simulink model "Model_aircraft_simple"  (R2024b)
settings: Solver=ode45  StartTime=0.0  StopTime=T_fin  RelTol=1e-10  EnableMultiTasking=on
values from neighbouring files (symbols this model uses):
  Euler_0 = [0; 0; 0]    [Main_simple.m]    (also in Script_trim_AI.m = x_trim(7:9))
  g = 9.81    [Main_simple.m]
  pqr_0 = [0; 0; 0]    [Main_simple.m]
  Ref_altitude = 0    [Main_simple.m]
  rho_0 = 1.293    [Main_simple.m]
  Tot_mom_inertia = diag([0.0494,0.0583,0.1012])    [Main_simple.m]
  Total_mass = 0.573    [Main_simple.m]
  u_0 = [0; 0; 0; 0]    [Main_simple.m]    (also in Script_trim_AI.m = u_0+u_trim)
  uvw_0 = [12.37 ;0; 0]    [Main_simple.m]    (also in Script_trim_AI.m = x_trim(4:6))
libraries: Library_simple_model x7
settings Model: Creator=Drago  LastModifiedBy=gregor
settings SolverCC: AlgebraicLoopSolver=TrustRegion
settings DataIOCC: LimitDataPoints=on  SaveFormat=Array
settings OptimizationCC: LifeSpan=inf
settings DebuggingCC: UnconnectedInputMsg=warning  UnconnectedOutputMsg=warning  UnconnectedLineMsg=warning  InitInArrayFormatMsg=none  SFUnexpectedBacktrackingDiag=warning  SFNoUnconditionalDefaultTransitionDiag=warning  SFExecutionAtInitializationDiag=none  ArithmeticOperatorsInVariantConditions=warning
settings HardwareCC: ProdBitPerPointer=32  ProdBitPerSizeT=32  ProdBitPerPtrDiffT=32  ProdLargestAtomicFloat=None  ProdIntDivRoundTo=Undefined  ProdEndianess=Unspecified  ProdWordSize=32  ProdHWDeviceType=32-bit Generic
settings ModelReferenceCC: EnableRefExpFcnMdlSchedulingChecks=on  PropagateSignalLabelsOutOfModel=off
settings SFSimCC: SimUseLocalCustomCode=off  CustomCodeUndefinedFunction=UseInterfaceOnly
settings RTWCC: RTWUseLocalCustomCode=off  GPUComputeCapability=3.5  DLArmComputeVersion=19.05
settings CodeAppCC: StateflowObjectComments=on
settings GRTTargetCC: TargetLangStandard=C89/C90 (ANSI)
settings ConfigComp: CovMetricSettings=dw  CovSaveCumulativeToWorkspaceVar=on  CovSaveSingleToWorkspaceVar=on  CovExternalEMLEnable=off  CovSFcnEnable=off

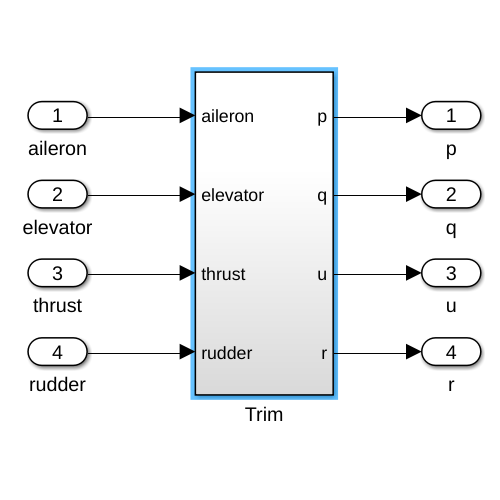
[thumbnail: Simulink's stored preview of the top-level diagram]
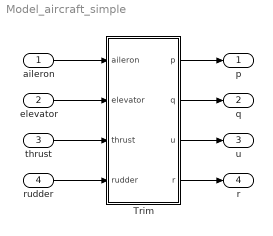
== system Model_aircraft_simple ==
  aileron : Inport
  elevator : Inport  Port=2
  thrust : Inport  Port=3
  rudder : Inport  Port=4
  Trim : Subsystem
  p : Outport
  q : Outport  Port=2
  u : Outport  Port=3
  r : Outport  Port=4
  wires:
  aileron/1 -> Trim/1(aileron)
  elevator/1 -> Trim/2(elevator)
  thrust/1 -> Trim/3(thrust)
  rudder/1 -> Trim/4(rudder)
  Trim/1(p) -> p/1
  Trim/2(q) -> q/1
  Trim/3(u) -> u/1
  Trim/4(r) -> r/1

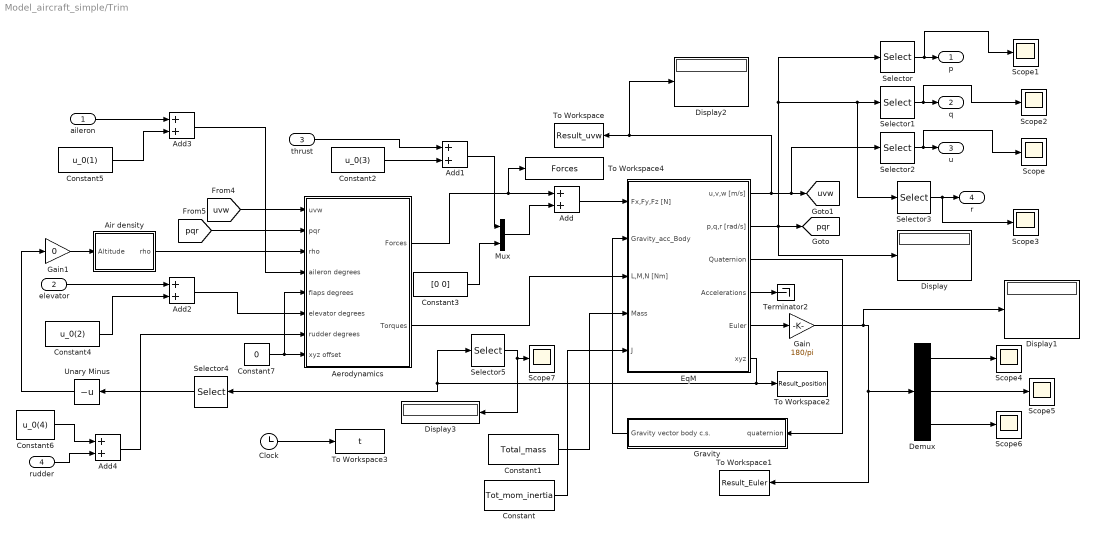
== system Model_aircraft_simple/Trim ==
  aileron : Inport
  elevator : Inport  Port=2
  thrust : Inport  Port=3
  rudder : Inport  Port=4
  Add{,1..4} (5 alike) : Sum
  "Aerodynamics " : Subsystem
  Air density : Subsystem
  Clock : Clock
  Constant : Constant  Value=Tot_mom_inertia
  Constant1 : Constant  Value=Total_mass
  Constant2 : Constant  Value=u_0(3)
  Constant3 : Constant  Value=[0 0]
  Constant4 : Constant  Value=u_0(2)
  Constant5 : Constant  Value=u_0(1)
  Constant6 : Constant  Value=u_0(4)
  Constant7 : Constant  Value=0
  Demux : Demux  Outputs=3
  Display{,1..3} (4 alike) : Display
  EqM : Subsystem
  Gain : Gain  Gain=180/pi
  Gain1 : Gain  Gain=0
  Gravity : Subsystem
  Mux : Mux  Inputs=2
  Scope{,1..7} (8 alike) : Scope
  Selector : Selector  InputPortWidth=3  IndexOptions=Index vector (dialog)  Indices=1  OutputSizes=1
  Selector1 : Selector  InputPortWidth=3  IndexOptions=Index vector (dialog)  Indices=2  OutputSizes=1
  Selector2 : Selector  InputPortWidth=3  IndexOptions=Index vector (dialog)  Indices=1  OutputSizes=1
  Selector3 : Selector  InputPortWidth=3  IndexOptions=Index vector (dialog)  Indices=3  OutputSizes=1
  Selector4 : Selector  InputPortWidth=3  IndexOptions=Index vector (dialog)  Indices=3  OutputSizes=1
  Selector5 : Selector  InputPortWidth=3  IndexOptions=Index vector (dialog)  Indices=3  OutputSizes=1
  Terminator2 : Terminator
  To Workspace : ToWorkspace  VariableName=Result_uvw  SampleTime=0.2
  To Workspace1 : ToWorkspace  VariableName=Result_Euler  SampleTime=0.2
  To Workspace2 : ToWorkspace  VariableName=Result_position  SampleTime=0.2
  To Workspace3 : ToWorkspace  VariableName=t  SampleTime=0.2
  To Workspace4 : ToWorkspace  VariableName=Forces  SampleTime=0.2
  Unary Minus : UnaryMinus
  p : Outport
  q : Outport  Port=2
  u : Outport  Port=3
  r : Outport  Port=4
  tag scope: pqr=global, uvw=global
  wires:
  Add1/1 -> Mux/1
  Gain/1 -> Display1/1, Demux/1, To Workspace1/1
  EqM/4(Accelerations) -> Terminator2/1
  Air density/1(rho) -> "Aerodynamics "/3(rho)
  EqM/2(p,q,r [rad/s]) -> Display/1, Selector3/1, Selector1/1, Selector/1, [pqr]
  Gravity/1(Gravity vector body c.s.) -> EqM/2(Gravity_acc_Body)
  EqM/3(Quaternion) -> Gravity/1(quaternion)
  [uvw] -> "Aerodynamics "/1(uvw)
  Add/1 -> EqM/1(Fx,Fy,Fz [N])
  "Aerodynamics "/2(Torques) -> EqM/3(L,M,N [Nm])
  "Aerodynamics "/1(Forces) -> To Workspace4/1, Add/1
  Constant1/1 -> EqM/4(Mass)
  EqM/1(u,v,w [m/s]) -> Display2/1, To Workspace/1, Selector2/1, [uvw]
  Constant/1 -> EqM/5(J)
  [pqr] -> "Aerodynamics "/2(pqr)
  EqM/5(Euler) -> Gain/1
  Constant3/1 -> Mux/2
  rudder/1 -> Add4/2
  Selector4/1 -> Unary Minus/1
  Mux/1 -> Add/2
  Add3/1 -> "Aerodynamics "/4(aileron degrees)
  Constant2/1 -> Add1/2
  aileron/1 -> Add3/1
  elevator/1 -> Add2/1
  Constant4/1 -> Add2/2
  Constant5/1 -> Add3/2
  Add4/1 -> "Aerodynamics "/7(rudder degrees)
  thrust/1 -> Add1/1
  Add2/1 -> "Aerodynamics "/6(elevator degrees)
  EqM/6(xyz) -> Selector4/1, Selector5/1, To Workspace2/1
  Constant6/1 -> Add4/1
  Clock/1 -> To Workspace3/1
  Constant7/1 -> "Aerodynamics "/5(flaps degrees), "Aerodynamics "/8(xyz offset)
  Selector/1 -> Scope1/1, p/1
  Selector1/1 -> Scope2/1, q/1
  Selector2/1 -> Scope/1, u/1
  Selector3/1 -> Scope3/1, r/1
  Unary Minus/1 -> Gain1/1
  Demux/1 -> Scope4/1
  Demux/2 -> Scope5/1
  Demux/3 -> Scope6/1
  Selector5/1 -> Display3/1, Scope7/1
  Gain1/1 -> Air density/1(Altitude)

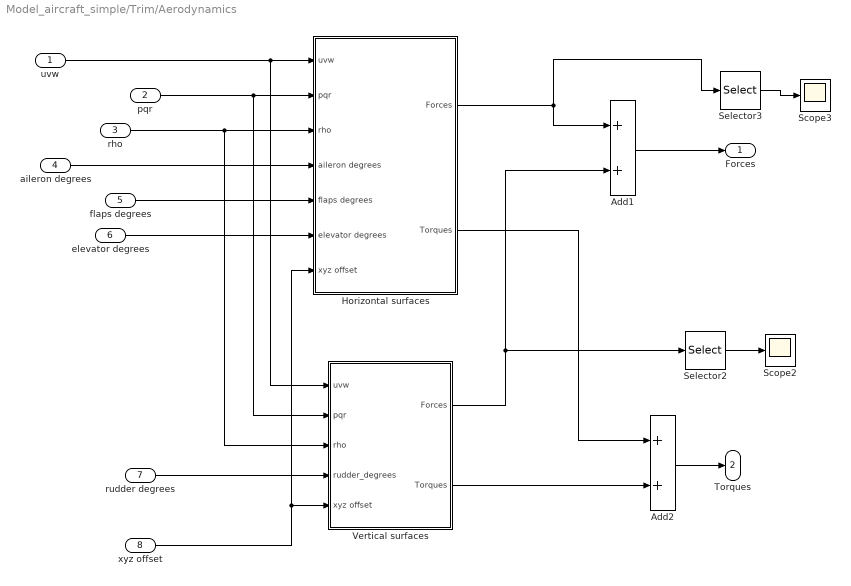
== system Model_aircraft_simple/Trim/Aerodynamics  ==
  uvw : Inport
  pqr : Inport  Port=2
  rho : Inport  Port=3
  aileron degrees : Inport  Port=4
  flaps degrees : Inport  Port=5
  elevator degrees : Inport  Port=6
  rudder degrees : Inport  Port=7
  xyz offset : Inport  Port=8
  Add1 : Sum
  Add2 : Sum
  Horizontal surfaces : Subsystem
  Scope2 : Scope
  Scope3 : Scope
  Selector2 : Selector  InputPortWidth=3  IndexOptions=Index vector (dialog)  Indices=[1 ]  OutputSizes=1
  Selector3 : Selector  InputPortWidth=3  IndexOptions=Index vector (dialog)  Indices=[1 ]  OutputSizes=1
  Vertical surfaces : Subsystem
  Forces : Outport
  Torques : Outport  Port=2
  wires:
  elevator degrees/1 -> Horizontal surfaces/6(elevator degrees)
  aileron degrees/1 -> Horizontal surfaces/4(aileron degrees)
  xyz offset/1 -> Horizontal surfaces/7(xyz offset), Vertical surfaces/5(xyz offset)
  rho/1 -> Vertical surfaces/3(rho), Horizontal surfaces/3(rho)
  pqr/1 -> Vertical surfaces/2(pqr), Horizontal surfaces/2(pqr)
  flaps degrees/1 -> Horizontal surfaces/5(flaps degrees)
  uvw/1 -> Vertical surfaces/1(uvw), Horizontal surfaces/1(uvw)
  Add2/1 -> Torques/1
  Horizontal surfaces/1(Forces) -> Selector3/1, Add1/1
  Add1/1 -> Forces/1
  Vertical surfaces/1(Forces) -> Selector2/1, Add1/2
  Horizontal surfaces/2(Torques) -> Add2/1
  rudder degrees/1 -> Vertical surfaces/4(rudder_degrees)
  Vertical surfaces/2(Torques) -> Add2/2
  Selector2/1 -> Scope2/1
  Selector3/1 -> Scope3/1

== system Model_aircraft_simple/Trim/Air density ==
  Altitude : Inport
  Gain : Gain  Gain=rho_0
  exp(-h/8000) : Fcn  Expr=exp(-u(1)/8000)
  rho : Outport
  wires:
  Gain/1 -> rho/1
  Altitude/1 -> exp(-h/8000)/1
  exp(-h/8000)/1 -> Gain/1

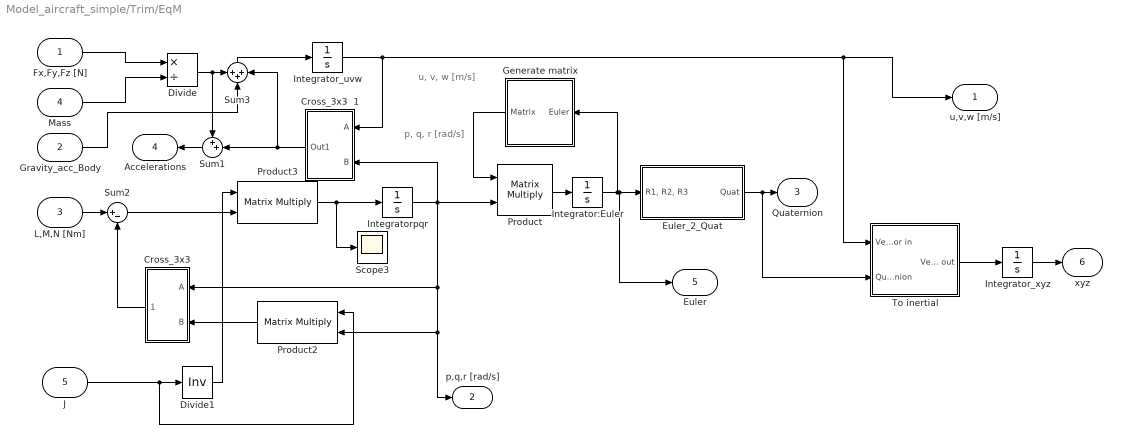
== system Model_aircraft_simple/Trim/EqM ==
  note: u, v, w [m/s]
  note: p, q, r [rad/s]
  Fx,Fy,Fz [N] : Inport
  Gravity_acc_Body : Inport  Port=2
  L,M,N [Nm] : Inport  Port=3
  Mass : Inport  Port=4
  J : Inport  Port=5
  Cross_3x3 : Subsystem
  Cross_3x3  1 : Subsystem
  Divide : Product  Inputs=*/
  Divide1 : Product  Inputs=/  Multiplication=Matrix(*)
  Euler_2_Quat : Subsystem
  Generate matrix : Subsystem
  Integrator:Euler : Integrator  InitialCondition=Euler_0  ZeroCross=off
  Integrator_uvw : Integrator  InitialCondition=uvw_0  ZeroCross=off
  Integrator_xyz : Integrator  InitialCondition=[0 0 -Ref_altitude]  ZeroCross=off
  Integratorpqr : Integrator  InitialCondition=pqr_0  ZeroCross=off
  Product : Product  Multiplication=Matrix(*)
  Product2 : Product  Multiplication=Matrix(*)
  Product3 : Product  Multiplication=Matrix(*)
  Scope3 : Scope
  Sum1 : Sum  Inputs=++|
  Sum2 : Sum  Inputs=|+-
  Sum3 : Sum  Inputs=+++
  To inertial : Subsystem
  u,v,w [m/s] : Outport
  p,q,r [rad/s] : Outport  Port=2
  Quaternion : Outport  Port=3
  Accelerations : Outport  Port=4
  Euler : Outport  Port=5
  xyz : Outport  Port=6
  wires:
  L,M,N [Nm]/1 -> Sum2/1
  Fx,Fy,Fz [N]/1 -> Divide/1
  Euler_2_Quat/1(Quat) -> To inertial/2(Quaternion), Quaternion/1
  Product2/1 -> Cross_3x3/2(B)
  Product3/1 -> Scope3/1, Integratorpqr/1
  Sum2/1 -> Product3/2
  Sum3/1 -> Integrator_uvw/1
  Integrator_uvw/1 -> Cross_3x3  1/1(A), To inertial/1(Vector in), u,v,w [m/s]/1
  Integratorpqr/1 -> Product/2, Cross_3x3  1/2(B), Product2/2, p,q,r [rad/s]/1, Cross_3x3/1(A)
  Cross_3x3/1(Out1) -> Sum2/2
  Cross_3x3  1/1(Out1) -> Sum3/3, Sum1/2
  Gravity_acc_Body/1 -> Sum3/2
  Divide/1 -> Sum1/1, Sum3/1
  Sum1/1 -> Accelerations/1
  Mass/1 -> Divide/2
  J/1 -> Product2/1, Divide1/1
  Divide1/1 -> Product3/1
  To inertial/1(Vector out) -> Integrator_xyz/1
  Integrator_xyz/1 -> xyz/1
  Product/1 -> Integrator:Euler/1
  Generate matrix/1(Matrix) -> Product/1
  Integrator:Euler/1 -> Generate matrix/1("Euler "), Euler_2_Quat/1("R1, R2, R3"), Euler/1

== system Model_aircraft_simple/Trim/Gravity ==
  quaternion : Inport
  Gravitational force : Constant  Value=[0 0 g]
  Inertial_2_body1 : Subsystem
  Gravity vector body c.s. : Outport
  wires:
  Gravitational force/1 -> Inertial_2_body1/1(Vector in)
  quaternion/1 -> Inertial_2_body1/2(Quaternion)
  Inertial_2_body1/1(Vector out) -> Gravity vector body c.s./1

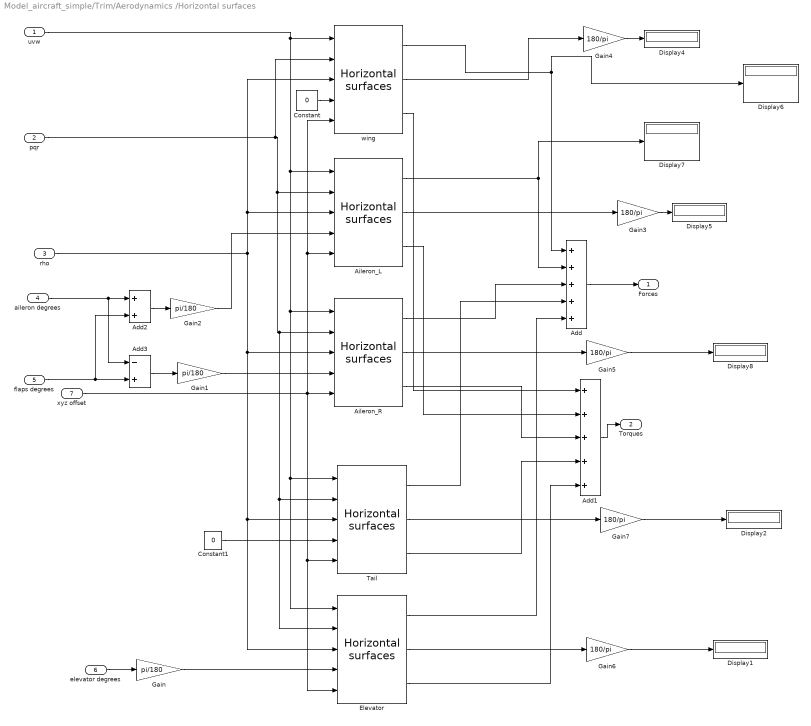
== system Model_aircraft_simple/Trim/Aerodynamics /Horizontal surfaces ==
  uvw : Inport
  pqr : Inport  Port=2
  rho : Inport  Port=3
  aileron degrees : Inport  Port=4
  flaps degrees : Inport  Port=5
  elevator degrees : Inport  Port=6
  xyz offset : Inport  Port=7
  Add : Sum  Inputs=+++++
  Add1 : Sum  Inputs=+++++
  Add2 : Sum
  Add3 : Sum  Inputs=-+
  Aileron_L : Library_simple_model/Horizontal surfaces  xyz_Aero=xyz_aileron_L  S_Wing=S__aileron_L  Alpha_0=Alpha_0_aileron_L  Alpha_param_Vector=Alpha_param_vector_aileron_L  CL_param_Vector=CL_param_vector_aileron_L  CD_param_Vector=CD_param_vector_aileron_L
  Aileron_R : Library_simple_model/Horizontal surfaces  xyz_Aero=xyz_aileron_R  S_Wing=S__aileron_R  Alpha_0=Alpha_0_aileron_R  Alpha_param_Vector=Alpha_param_vector_aileron_R  CL_param_Vector=CL_param_vector_aileron_R  CD_param_Vector=CD_param_vector_aileron_R
  Constant : Constant  Value=0
  Constant1 : Constant  Value=0
  Display{1..2,4..8} (7 alike) : Display
  Elevator : Library_simple_model/Horizontal surfaces  xyz_Aero=xyz_elevator  S_Wing=S_elevator  Alpha_0=Alpha_0_elevator  Alpha_param_Vector=Alpha_param_vector_elevator  CL_param_Vector=CL_param_vector_elevator  CD_param_Vector=CD_param_vector_elevator
  Gain : Gain  Gain=pi/180
  Gain1 : Gain  Gain=pi/180
  Gain2 : Gain  Gain=pi/180
  Gain{3..7} (5 alike) : Gain  Gain=180/pi
  Tail : Library_simple_model/Horizontal surfaces  xyz_Aero=xyz_horiz_stabilizer  S_Wing=S_horiz_stabilizer  Alpha_0=Alpha_0_horiz_stabilizer  Alpha_param_Vector=Alpha_param_vector_horiz_stabilizer  CL_param_Vector=CL_param_vector_horiz_stabilizer  CD_param_Vector=CD_param_vector_horiz_stabilizer
  wing : Library_simple_model/Horizontal surfaces  xyz_Aero=xyz_wing  S_Wing=S_wing  Alpha_0=Alpha_0_wing  Alpha_param_Vector=Alpha_param_vector_wing  CL_param_Vector=CL_param_vector_wing  CD_param_Vector=CD_param_vector_wing
  Forces : Outport
  Torques : Outport  Port=2
  wires:
  Add1/1 -> Torques/1
  Aileron_R/3 -> Add1/3
  wing/3 -> Add1/1
  pqr/1 -> wing/2, Elevator/2, Tail/2, Aileron_R/2, Aileron_L/2
  aileron degrees/1 -> Add3/1, Add2/1
  elevator degrees/1 -> Gain/1
  Aileron_L/1 -> Display7/1, Add/2
  wing/1 -> Display6/1, Add/1
  Aileron_R/1 -> Add/3
  rho/1 -> Elevator/3, Tail/3, Aileron_R/3, Aileron_L/3, wing/3
  uvw/1 -> wing/1, Elevator/1, Tail/1, Aileron_R/1, Aileron_L/1
  Gain1/1 -> Aileron_R/4
  Add3/1 -> Gain1/1
  Gain2/1 -> Aileron_L/4
  flaps degrees/1 -> Add2/2, Add3/2
  Add2/1 -> Gain2/1
  Add/1 -> Forces/1
  Aileron_L/3 -> Add1/2
  xyz offset/1 -> Elevator/5, Tail/5, Aileron_R/5, Aileron_L/5, wing/5
  wing/2 -> Gain4/1
  Aileron_L/2 -> Gain3/1
  Gain3/1 -> Display5/1
  Gain4/1 -> Display4/1
  Aileron_R/2 -> Gain5/1
  Gain5/1 -> Display8/1
  Constant/1 -> wing/4
  Tail/3 -> Add1/4
  Tail/1 -> Add/4
  Gain/1 -> Elevator/4
  Constant1/1 -> Tail/4
  Elevator/3 -> Add1/5
  Elevator/1 -> Add/5
  Gain6/1 -> Display1/1
  Elevator/2 -> Gain6/1
  Gain7/1 -> Display2/1
  Tail/2 -> Gain7/1

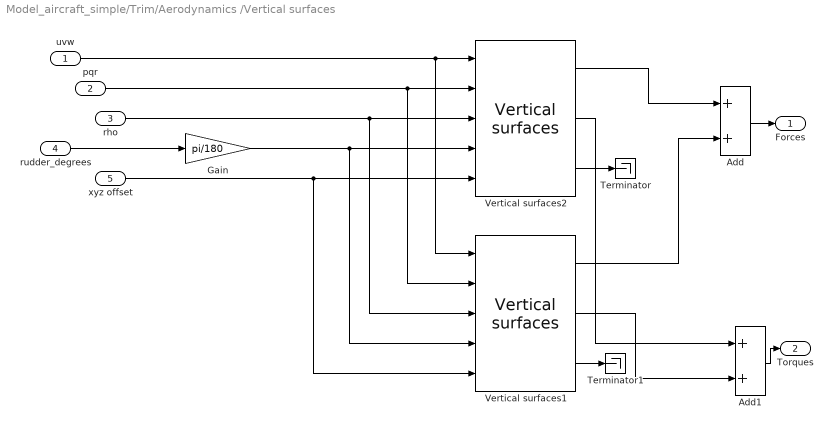
== system Model_aircraft_simple/Trim/Aerodynamics /Vertical surfaces ==
  uvw : Inport
  pqr : Inport  Port=2
  rho : Inport  Port=3
  rudder_degrees : Inport  Port=4
  xyz offset : Inport  Port=5
  Add : Sum
  Add1 : Sum
  Gain : Gain  Gain=pi/180
  Terminator : Terminator
  Terminator1 : Terminator
  Vertical surfaces1 : Library_simple_model/Vertical surfaces  xyzbody_Vert_stab=xyz_rudder  S_Body_Vert_stab=S_rudder  beta_param_Vert_stab_param=Beta_param_vector_rudder  CY_Vert_stab_param=CY_param_vector_rudder  CD_Vert_stab_param=CD_param_vector_rudder
  Vertical surfaces2 : Library_simple_model/Vertical surfaces  xyzbody_Vert_stab=xyz_vert_stabilizer  S_Body_Vert_stab=S_vert_stabilizer  beta_param_Vert_stab_param=Beta_param_vector_vert_stabilizer  CY_Vert_stab_param=CY_param_vector_vert_stabilizer  CD_Vert_stab_param=CD_param_vector_vert_stabilizer
  Forces : Outport
  Torques : Outport  Port=2
  wires:
  pqr/1 -> Vertical surfaces1/2, Vertical surfaces2/2
  rho/1 -> Vertical surfaces1/3, Vertical surfaces2/3
  Vertical surfaces2/3 -> Terminator/1
  xyz offset/1 -> Vertical surfaces1/5, Vertical surfaces2/5
  rudder_degrees/1 -> Gain/1
  uvw/1 -> Vertical surfaces1/1, Vertical surfaces2/1
  Vertical surfaces1/3 -> Terminator1/1
  Add1/1 -> Torques/1
  Vertical surfaces2/1 -> Add/1
  Vertical surfaces1/1 -> Add/2
  Vertical surfaces2/2 -> Add1/1
  Vertical surfaces1/2 -> Add1/2
  Add/1 -> Forces/1
  Gain/1 -> Vertical surfaces1/4, Vertical surfaces2/4

== system Model_aircraft_simple/Trim/EqM/Cross_3x3 ==
  A : Inport
  B : Inport  Port=2
  Subsystem : Subsystem
  Subsystem1 : Subsystem
  Sum2 : Sum  Inputs=+|-  InputSameDT=on  SaturateOnIntegerOverflow=on  OutDataTypeStr=Inherit: Same as first input
  Out1 : Outport
  wires:
  B/1 -> Subsystem/2(B1), Subsystem1/2(B1)
  Subsystem1/1(Out2) -> Sum2/2
  Subsystem/1(Out2) -> Sum2/1
  Sum2/1 -> Out1/1
  A/1 -> Subsystem1/1(A1), Subsystem/1(A1)

== system Model_aircraft_simple/Trim/EqM/Cross_3x3  1 ==
  A : Inport
  B : Inport  Port=2
  Subsystem : Subsystem
  Subsystem1 : Subsystem
  Sum2 : Sum  Inputs=+|-  InputSameDT=on  SaturateOnIntegerOverflow=on  OutDataTypeStr=Inherit: Same as first input
  Out1 : Outport
  wires:
  B/1 -> Subsystem/2(B1), Subsystem1/2(B1)
  Subsystem1/1(Out2) -> Sum2/2
  Subsystem/1(Out2) -> Sum2/1
  Sum2/1 -> Out1/1
  A/1 -> Subsystem1/1(A1), Subsystem/1(A1)

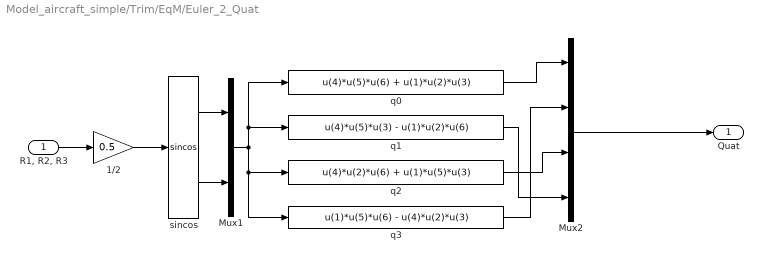
== system Model_aircraft_simple/Trim/EqM/Euler_2_Quat ==
  "R1, R2, R3" : Inport
  1/2 : Gain  Gain=0.5  SaturateOnIntegerOverflow=on  OutDataTypeStr=Inherit: Same as input  ParamDataTypeStr=Inherit: Same as input
  Mux1 : Mux  Inputs=2
  Mux2 : Mux
  q0 : Fcn  Expr=u(4)*u(5)*u(6) + u(1)*u(2)*u(3)
  q1 : Fcn  Expr=u(4)*u(5)*u(3) - u(1)*u(2)*u(6)
  q2 : Fcn  Expr=u(4)*u(2)*u(6) + u(1)*u(5)*u(3)
  q3 : Fcn  Expr=u(1)*u(5)*u(6) - u(4)*u(2)*u(3)
  sincos : Trigonometry  Operator=sincos
  Quat : Outport  InitialOutput=0
  wires:
  q1/1 -> Mux2/4
  sincos/2 -> Mux1/2
  q2/1 -> Mux2/3
  sincos/1 -> Mux1/1
  q0/1 -> Mux2/1
  Mux1/1 -> q0/1, q1/1, q2/1, q3/1
  1/2/1 -> sincos/1
  Mux2/1 -> Quat/1
  q3/1 -> Mux2/2
  "R1, R2, R3"/1 -> 1/2/1

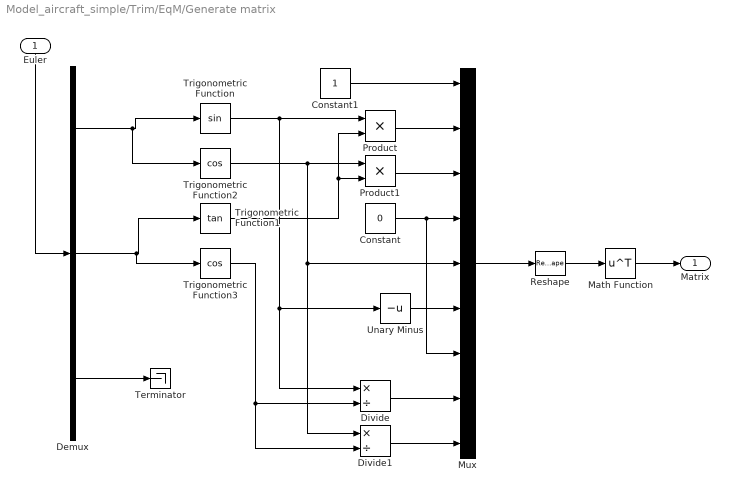
== system Model_aircraft_simple/Trim/EqM/Generate matrix ==
  "Euler " : Inport
  Constant : Constant  Value=0
  Constant1 : Constant
  Demux : Demux  Outputs=3
  Divide : Product  Inputs=*/
  Divide1 : Product  Inputs=*/
  Math Function : Math  Operator=transpose  SignedPower=on
  Mux : Mux  Inputs=9
  Product : Product
  Product1 : Product
  Reshape : Reshape  OutputDimensionality=Customize  OutputDimensions=[3,3]
  Terminator : Terminator
  Trigonometric Function : Trigonometry
  Trigonometric Function1 : Trigonometry  Operator=tan
  Trigonometric Function2 : Trigonometry  Operator=cos
  Trigonometric Function3 : Trigonometry  Operator=cos
  Unary Minus : UnaryMinus
  Matrix : Outport
  wires:
  Demux/1 -> Trigonometric Function2/1, Trigonometric Function/1
  Demux/3 -> Terminator/1
  "Euler "/1 -> Demux/1
  Demux/2 -> Trigonometric Function3/1, Trigonometric Function1/1
  Mux/1 -> Reshape/1
  Product/1 -> Mux/2
  Trigonometric Function/1 -> Divide/1, Unary Minus/1, Product/1
  Trigonometric Function1/1 -> Product1/2, Product/2
  Product1/1 -> Mux/3
  Trigonometric Function2/1 -> Divide1/1, Mux/5, Product1/1
  Unary Minus/1 -> Mux/6
  Constant/1 -> Mux/7, Mux/4
  Divide/1 -> Mux/8
  Divide1/1 -> Mux/9
  Trigonometric Function3/1 -> Divide/2, Divide1/2
  Reshape/1 -> Math Function/1
  Constant1/1 -> Mux/1
  Math Function/1 -> Matrix/1

== system Model_aircraft_simple/Trim/EqM/To inertial ==
  note: To inertial
  Vector in : Inport
  Quaternion : Inport  Port=2
  Conjugate quaternion : Subsystem
  Product of quaternions1 : Subsystem
  Product of quaternions2 : Subsystem
  Quaternion _2_vector : Subsystem
  Vector_2_ quaternion : Subsystem
  Vector out : Outport
  wires:
  Product of quaternions2/1(Out1) -> Product of quaternions1/1(In1)
  Vector_2_ quaternion/1(Out1) -> Product of quaternions2/2(In2)
  Conjugate quaternion/1(Out1) -> Product of quaternions1/2(In2)
  Product of quaternions1/1(Out1) -> Quaternion _2_vector/1(In1)
  Vector in/1 -> Vector_2_ quaternion/1(In1)
  Quaternion/1 -> Conjugate quaternion/1(In1), Product of quaternions2/1(In1)
  Quaternion _2_vector/1(Out1) -> Vector out/1

== system Model_aircraft_simple/Trim/Gravity/Inertial_2_body1 ==
  Vector in : Inport
  Quaternion : Inport  Port=2
  Conjugate quaternion : Subsystem
  Product of quaternions1 : Subsystem
  Product of quaternions2 : Subsystem
  Quaternion _2_vector : Subsystem
  Vector_2_ quaternion : Subsystem
  Vector out : Outport
  wires:
  Product of quaternions2/1(Out1) -> Product of quaternions1/1(In1)
  Vector_2_ quaternion/1(Out1) -> Product of quaternions2/2(In2)
  Product of quaternions1/1(Out1) -> Quaternion _2_vector/1(In1)
  Vector in/1 -> Vector_2_ quaternion/1(In1)
  Quaternion/1 -> Conjugate quaternion/1(In1), Product of quaternions1/2(In2)
  Quaternion _2_vector/1(Out1) -> Vector out/1
  Conjugate quaternion/1(Out1) -> Product of quaternions2/1(In1)

== system Model_aircraft_simple/Trim/EqM/Cross_3x3/Subsystem ==
  A1 : Inport
  B1 : Inport  Port=2
  Demux : Demux  Outputs=3
  Demux1 : Demux  Outputs=3
  Mux : Mux  Inputs=3
  i x j : Product  InputSameDT=on  SaturateOnIntegerOverflow=on  OutDataTypeStr=Inherit: Same as first input
  j x k : Product  InputSameDT=on  SaturateOnIntegerOverflow=on  OutDataTypeStr=Inherit: Same as first input
  k x i : Product  InputSameDT=on  SaturateOnIntegerOverflow=on  OutDataTypeStr=Inherit: Same as first input
  Out2 : Outport
  wires:
  k x i/1 -> Mux/2
  Demux1/2 -> i x j/2
  Demux1/3 -> j x k/2
  Demux1/1 -> k x i/2
  Demux/3 -> k x i/1
  Mux/1 -> Out2/1
  Demux/2 -> j x k/1
  j x k/1 -> Mux/1
  i x j/1 -> Mux/3
  B1/1 -> Demux1/1
  Demux/1 -> i x j/1
  A1/1 -> Demux/1

== system Model_aircraft_simple/Trim/EqM/Cross_3x3/Subsystem1 ==
  A1 : Inport
  B1 : Inport  Port=2
  Demux : Demux  Outputs=3
  Demux1 : Demux  Outputs=3
  Mux : Mux  Inputs=3
  i x k : Product  InputSameDT=on  SaturateOnIntegerOverflow=on  OutDataTypeStr=Inherit: Same as first input
  j x i : Product  InputSameDT=on  SaturateOnIntegerOverflow=on  OutDataTypeStr=Inherit: Same as first input
  k x j : Product  InputSameDT=on  SaturateOnIntegerOverflow=on  OutDataTypeStr=Inherit: Same as first input
  Out2 : Outport
  wires:
  j x i/1 -> Mux/3
  i x k/1 -> Mux/2
  k x j/1 -> Mux/1
  Mux/1 -> Out2/1
  Demux1/1 -> j x i/2
  Demux/2 -> j x i/1
  Demux1/3 -> i x k/2
  Demux/1 -> i x k/1
  Demux/3 -> k x j/1
  Demux1/2 -> k x j/2
  B1/1 -> Demux1/1
  A1/1 -> Demux/1

== system Model_aircraft_simple/Trim/EqM/Cross_3x3  1/Subsystem ==
  A1 : Inport
  B1 : Inport  Port=2
  Demux : Demux  Outputs=3
  Demux1 : Demux  Outputs=3
  Mux : Mux  Inputs=3
  i x j : Product  InputSameDT=on  SaturateOnIntegerOverflow=on  OutDataTypeStr=Inherit: Same as first input
  j x k : Product  InputSameDT=on  SaturateOnIntegerOverflow=on  OutDataTypeStr=Inherit: Same as first input
  k x i : Product  InputSameDT=on  SaturateOnIntegerOverflow=on  OutDataTypeStr=Inherit: Same as first input
  Out2 : Outport
  wires:
  k x i/1 -> Mux/2
  Demux1/2 -> i x j/2
  Demux1/3 -> j x k/2
  Demux1/1 -> k x i/2
  Demux/3 -> k x i/1
  Mux/1 -> Out2/1
  Demux/2 -> j x k/1
  j x k/1 -> Mux/1
  i x j/1 -> Mux/3
  B1/1 -> Demux1/1
  Demux/1 -> i x j/1
  A1/1 -> Demux/1

== system Model_aircraft_simple/Trim/EqM/Cross_3x3  1/Subsystem1 ==
  A1 : Inport
  B1 : Inport  Port=2
  Demux : Demux  Outputs=3
  Demux1 : Demux  Outputs=3
  Mux : Mux  Inputs=3
  i x k : Product  InputSameDT=on  SaturateOnIntegerOverflow=on  OutDataTypeStr=Inherit: Same as first input
  j x i : Product  InputSameDT=on  SaturateOnIntegerOverflow=on  OutDataTypeStr=Inherit: Same as first input
  k x j : Product  InputSameDT=on  SaturateOnIntegerOverflow=on  OutDataTypeStr=Inherit: Same as first input
  Out2 : Outport
  wires:
  j x i/1 -> Mux/3
  i x k/1 -> Mux/2
  k x j/1 -> Mux/1
  Mux/1 -> Out2/1
  Demux1/1 -> j x i/2
  Demux/2 -> j x i/1
  Demux1/3 -> i x k/2
  Demux/1 -> i x k/1
  Demux/3 -> k x j/1
  Demux1/2 -> k x j/2
  B1/1 -> Demux1/1
  A1/1 -> Demux/1

== system Model_aircraft_simple/Trim/EqM/To inertial/Conjugate quaternion ==
  In1 : Inport
  Demux1 : Demux
  Mux1 : Mux
  Unary Minus1 : UnaryMinus
  Unary Minus2 : UnaryMinus
  Unary Minus3 : UnaryMinus
  Out1 : Outport
  wires:
  Demux1/1 -> Mux1/1
  Unary Minus1/1 -> Mux1/2
  Unary Minus2/1 -> Mux1/3
  Unary Minus3/1 -> Mux1/4
  Demux1/2 -> Unary Minus1/1
  Demux1/3 -> Unary Minus2/1
  Demux1/4 -> Unary Minus3/1
  In1/1 -> Demux1/1
  Mux1/1 -> Out1/1

== system Model_aircraft_simple/Trim/EqM/To inertial/Product of quaternions1 ==
  In1 : Inport
  In2 : Inport  Port=2
  Mux : Mux
  q0 : Subsystem
  q1 : Subsystem
  q2 : Subsystem
  q3 : Subsystem
  Out1 : Outport
  wires:
  q0/1(q0) -> Mux/1
  q1/1(q1) -> Mux/2
  q2/1(q2) -> Mux/3
  q3/1(q3) -> Mux/4
  In1/1 -> q3/1(q), q2/1(q), q1/1(q), q0/1(q)
  In2/1 -> q1/2(r), q2/2(r), q3/2(r), q0/2(r)
  Mux/1 -> Out1/1

== system Model_aircraft_simple/Trim/EqM/To inertial/Product of quaternions2 ==
  In1 : Inport
  In2 : Inport  Port=2
  Mux : Mux
  q0 : Subsystem
  q1 : Subsystem
  q2 : Subsystem
  q3 : Subsystem
  Out1 : Outport
  wires:
  q0/1(q0) -> Mux/1
  q1/1(q1) -> Mux/2
  q2/1(q2) -> Mux/3
  q3/1(q3) -> Mux/4
  In1/1 -> q3/1(q), q2/1(q), q1/1(q), q0/1(q)
  In2/1 -> q1/2(r), q2/2(r), q3/2(r), q0/2(r)
  Mux/1 -> Out1/1

== system Model_aircraft_simple/Trim/EqM/To inertial/Quaternion _2_vector ==
  In1 : Inport
  Demux1 : Demux
  Mux1 : Mux  Inputs=3
  Terminator2 : Terminator
  Out1 : Outport
  wires:
  Demux1/2 -> Mux1/1
  Demux1/3 -> Mux1/2
  Demux1/4 -> Mux1/3
  Demux1/1 -> Terminator2/1
  In1/1 -> Demux1/1
  Mux1/1 -> Out1/1

== system Model_aircraft_simple/Trim/EqM/To inertial/Vector_2_ quaternion ==
  note: Vector_2_quaternion
  In1 : Inport
  Constant2 : Constant  Value=0
  Mux : Mux  Inputs=2
  Out1 : Outport
  wires:
  Constant2/1 -> Mux/1
  In1/1 -> Mux/2
  Mux/1 -> Out1/1

== system Model_aircraft_simple/Trim/Gravity/Inertial_2_body1/Conjugate quaternion ==
  In1 : Inport
  Demux1 : Demux
  Mux1 : Mux
  Unary Minus1 : UnaryMinus
  Unary Minus2 : UnaryMinus
  Unary Minus3 : UnaryMinus
  Out1 : Outport
  wires:
  Demux1/1 -> Mux1/1
  Unary Minus1/1 -> Mux1/2
  Unary Minus2/1 -> Mux1/3
  Unary Minus3/1 -> Mux1/4
  Demux1/2 -> Unary Minus1/1
  Demux1/3 -> Unary Minus2/1
  Demux1/4 -> Unary Minus3/1
  In1/1 -> Demux1/1
  Mux1/1 -> Out1/1

== system Model_aircraft_simple/Trim/Gravity/Inertial_2_body1/Product of quaternions1 ==
  In1 : Inport
  In2 : Inport  Port=2
  Mux : Mux
  q0 : Subsystem
  q1 : Subsystem
  q2 : Subsystem
  q3 : Subsystem
  Out1 : Outport
  wires:
  Mux/1 -> Out1/1
  In2/1 -> q0/2(r), q3/2(r), q2/2(r), q1/2(r)
  In1/1 -> q0/1(q), q1/1(q), q2/1(q), q3/1(q)
  q3/1(q3) -> Mux/4
  q2/1(q2) -> Mux/3
  q1/1(q1) -> Mux/2
  q0/1(q0) -> Mux/1

== system Model_aircraft_simple/Trim/Gravity/Inertial_2_body1/Product of quaternions2 ==
  In1 : Inport
  In2 : Inport  Port=2
  Mux : Mux
  q0 : Subsystem
  q1 : Subsystem
  q2 : Subsystem
  q3 : Subsystem
  Out1 : Outport
  wires:
  q0/1(q0) -> Mux/1
  q1/1(q1) -> Mux/2
  q2/1(q2) -> Mux/3
  q3/1(q3) -> Mux/4
  In1/1 -> q3/1(q), q2/1(q), q1/1(q), q0/1(q)
  In2/1 -> q1/2(r), q2/2(r), q3/2(r), q0/2(r)
  Mux/1 -> Out1/1

== system Model_aircraft_simple/Trim/Gravity/Inertial_2_body1/Quaternion _2_vector ==
  In1 : Inport
  Demux1 : Demux
  Mux1 : Mux  Inputs=3
  Terminator2 : Terminator
  Out1 : Outport
  wires:
  Demux1/2 -> Mux1/1
  Demux1/3 -> Mux1/2
  Demux1/4 -> Mux1/3
  Demux1/1 -> Terminator2/1
  In1/1 -> Demux1/1
  Mux1/1 -> Out1/1

== system Model_aircraft_simple/Trim/Gravity/Inertial_2_body1/Vector_2_ quaternion ==
  In1 : Inport
  Constant2 : Constant  Value=0
  Mux : Mux  Inputs=2
  Out1 : Outport
  wires:
  Constant2/1 -> Mux/1
  In1/1 -> Mux/2
  Mux/1 -> Out1/1

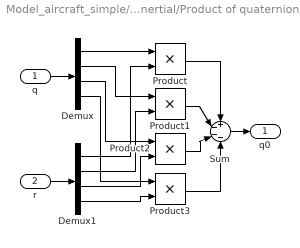
== system Model_aircraft_simple/Trim/EqM/To inertial/Product of quaternions1/q0 ==
  q : Inport
  r : Inport  Port=2
  Demux : Demux
  Demux1 : Demux
  Product{,1..3} (4 alike) : Product  RndMeth=Zero
  Sum : Sum  Inputs=+---
  q0 : Outport
  wires:
  q/1 -> Demux/1
  r/1 -> Demux1/1
  Demux/1 -> Product/1
  Demux1/1 -> Product/2
  Demux/2 -> Product1/1
  Demux1/2 -> Product1/2
  Demux/3 -> Product2/1
  Demux1/3 -> Product2/2
  Demux1/4 -> Product3/2
  Demux/4 -> Product3/1
  Product/1 -> Sum/1
  Product1/1 -> Sum/2
  Product3/1 -> Sum/4
  Sum/1 -> q0/1
  Product2/1 -> Sum/3

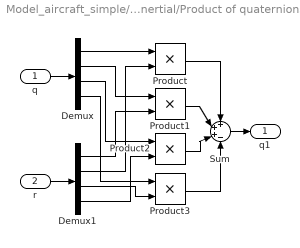
== system Model_aircraft_simple/Trim/EqM/To inertial/Product of quaternions1/q1 ==
  q : Inport
  r : Inport  Port=2
  Demux : Demux
  Demux1 : Demux
  Product{,1..3} (4 alike) : Product  RndMeth=Zero
  Sum : Sum  Inputs=+++-
  q1 : Outport
  wires:
  Product2/1 -> Sum/3
  Sum/1 -> q1/1
  Product3/1 -> Sum/4
  Product1/1 -> Sum/2
  Product/1 -> Sum/1
  Demux/4 -> Product3/1
  Demux/3 -> Product2/1
  Demux/2 -> Product1/1
  Demux/1 -> Product/1
  r/1 -> Demux1/1
  q/1 -> Demux/1
  Demux1/2 -> Product/2
  Demux1/1 -> Product1/2
  Demux1/4 -> Product2/2
  Demux1/3 -> Product3/2

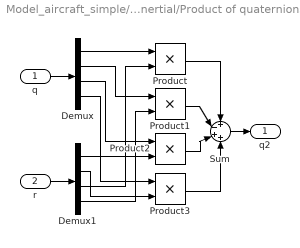
== system Model_aircraft_simple/Trim/EqM/To inertial/Product of quaternions1/q2 ==
  q : Inport
  r : Inport  Port=2
  Demux : Demux
  Demux1 : Demux
  Product{,1..3} (4 alike) : Product  RndMeth=Zero
  Sum : Sum  Inputs=+-++
  q2 : Outport
  wires:
  q/1 -> Demux/1
  r/1 -> Demux1/1
  Demux/1 -> Product/1
  Demux/2 -> Product1/1
  Demux/3 -> Product2/1
  Demux/4 -> Product3/1
  Product/1 -> Sum/1
  Product1/1 -> Sum/2
  Product3/1 -> Sum/4
  Sum/1 -> q2/1
  Product2/1 -> Sum/3
  Demux1/3 -> Product/2
  Demux1/4 -> Product1/2
  Demux1/1 -> Product2/2
  Demux1/2 -> Product3/2

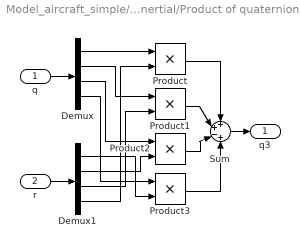
== system Model_aircraft_simple/Trim/EqM/To inertial/Product of quaternions1/q3 ==
  q : Inport
  r : Inport  Port=2
  Demux : Demux
  Demux1 : Demux
  Product{,1..3} (4 alike) : Product  RndMeth=Zero
  Sum : Sum  Inputs=++-+
  q3 : Outport
  wires:
  Product2/1 -> Sum/3
  Sum/1 -> q3/1
  Product3/1 -> Sum/4
  Product1/1 -> Sum/2
  Product/1 -> Sum/1
  Demux/4 -> Product3/1
  Demux/3 -> Product2/1
  Demux/2 -> Product1/1
  Demux/1 -> Product/1
  r/1 -> Demux1/1
  q/1 -> Demux/1
  Demux1/2 -> Product2/2
  Demux1/1 -> Product3/2
  Demux1/3 -> Product1/2
  Demux1/4 -> Product/2

== system Model_aircraft_simple/Trim/EqM/To inertial/Product of quaternions2/q0 ==
  q : Inport
  r : Inport  Port=2
  Demux : Demux
  Demux1 : Demux
  Product{,1..3} (4 alike) : Product  RndMeth=Zero
  Sum : Sum  Inputs=+---
  q0 : Outport
  wires:
  q/1 -> Demux/1
  r/1 -> Demux1/1
  Demux/1 -> Product/1
  Demux1/1 -> Product/2
  Demux/2 -> Product1/1
  Demux1/2 -> Product1/2
  Demux/3 -> Product2/1
  Demux1/3 -> Product2/2
  Demux1/4 -> Product3/2
  Demux/4 -> Product3/1
  Product/1 -> Sum/1
  Product1/1 -> Sum/2
  Product3/1 -> Sum/4
  Sum/1 -> q0/1
  Product2/1 -> Sum/3

== system Model_aircraft_simple/Trim/EqM/To inertial/Product of quaternions2/q1 ==
  q : Inport
  r : Inport  Port=2
  Demux : Demux
  Demux1 : Demux
  Product{,1..3} (4 alike) : Product  RndMeth=Zero
  Sum : Sum  Inputs=+++-
  q1 : Outport
  wires:
  Product2/1 -> Sum/3
  Sum/1 -> q1/1
  Product3/1 -> Sum/4
  Product1/1 -> Sum/2
  Product/1 -> Sum/1
  Demux/4 -> Product3/1
  Demux/3 -> Product2/1
  Demux/2 -> Product1/1
  Demux/1 -> Product/1
  r/1 -> Demux1/1
  q/1 -> Demux/1
  Demux1/2 -> Product/2
  Demux1/1 -> Product1/2
  Demux1/4 -> Product2/2
  Demux1/3 -> Product3/2

== system Model_aircraft_simple/Trim/EqM/To inertial/Product of quaternions2/q2 ==
  q : Inport
  r : Inport  Port=2
  Demux : Demux
  Demux1 : Demux
  Product{,1..3} (4 alike) : Product  RndMeth=Zero
  Sum : Sum  Inputs=+-++
  q2 : Outport
  wires:
  q/1 -> Demux/1
  r/1 -> Demux1/1
  Demux/1 -> Product/1
  Demux/2 -> Product1/1
  Demux/3 -> Product2/1
  Demux/4 -> Product3/1
  Product/1 -> Sum/1
  Product1/1 -> Sum/2
  Product3/1 -> Sum/4
  Sum/1 -> q2/1
  Product2/1 -> Sum/3
  Demux1/3 -> Product/2
  Demux1/4 -> Product1/2
  Demux1/1 -> Product2/2
  Demux1/2 -> Product3/2

== system Model_aircraft_simple/Trim/EqM/To inertial/Product of quaternions2/q3 ==
  q : Inport
  r : Inport  Port=2
  Demux : Demux
  Demux1 : Demux
  Product{,1..3} (4 alike) : Product  RndMeth=Zero
  Sum : Sum  Inputs=++-+
  q3 : Outport
  wires:
  Product2/1 -> Sum/3
  Sum/1 -> q3/1
  Product3/1 -> Sum/4
  Product1/1 -> Sum/2
  Product/1 -> Sum/1
  Demux/4 -> Product3/1
  Demux/3 -> Product2/1
  Demux/2 -> Product1/1
  Demux/1 -> Product/1
  r/1 -> Demux1/1
  q/1 -> Demux/1
  Demux1/2 -> Product2/2
  Demux1/1 -> Product3/2
  Demux1/3 -> Product1/2
  Demux1/4 -> Product/2

== system Model_aircraft_simple/Trim/Gravity/Inertial_2_body1/Product of quaternions1/q0 ==
  q : Inport
  r : Inport  Port=2
  Demux : Demux
  Demux1 : Demux
  Product{,1..3} (4 alike) : Product  RndMeth=Zero
  Sum : Sum  Inputs=+---
  q0 : Outport
  wires:
  Product2/1 -> Sum/3
  Sum/1 -> q0/1
  Product3/1 -> Sum/4
  Product1/1 -> Sum/2
  Product/1 -> Sum/1
  Demux/4 -> Product3/1
  Demux1/4 -> Product3/2
  Demux1/3 -> Product2/2
  Demux/3 -> Product2/1
  Demux1/2 -> Product1/2
  Demux/2 -> Product1/1
  Demux1/1 -> Product/2
  Demux/1 -> Product/1
  r/1 -> Demux1/1
  q/1 -> Demux/1

== system Model_aircraft_simple/Trim/Gravity/Inertial_2_body1/Product of quaternions1/q1 ==
  q : Inport
  r : Inport  Port=2
  Demux : Demux
  Demux1 : Demux
  Product{,1..3} (4 alike) : Product  RndMeth=Zero
  Sum : Sum  Inputs=+++-
  q1 : Outport
  wires:
  Demux1/3 -> Product3/2
  Demux1/4 -> Product2/2
  Demux1/1 -> Product1/2
  Demux1/2 -> Product/2
  q/1 -> Demux/1
  r/1 -> Demux1/1
  Demux/1 -> Product/1
  Demux/2 -> Product1/1
  Demux/3 -> Product2/1
  Demux/4 -> Product3/1
  Product/1 -> Sum/1
  Product1/1 -> Sum/2
  Product3/1 -> Sum/4
  Sum/1 -> q1/1
  Product2/1 -> Sum/3

== system Model_aircraft_simple/Trim/Gravity/Inertial_2_body1/Product of quaternions1/q2 ==
  q : Inport
  r : Inport  Port=2
  Demux : Demux
  Demux1 : Demux
  Product{,1..3} (4 alike) : Product  RndMeth=Zero
  Sum : Sum  Inputs=+-++
  q2 : Outport
  wires:
  Demux1/2 -> Product3/2
  Demux1/1 -> Product2/2
  Demux1/4 -> Product1/2
  Demux1/3 -> Product/2
  Product2/1 -> Sum/3
  Sum/1 -> q2/1
  Product3/1 -> Sum/4
  Product1/1 -> Sum/2
  Product/1 -> Sum/1
  Demux/4 -> Product3/1
  Demux/3 -> Product2/1
  Demux/2 -> Product1/1
  Demux/1 -> Product/1
  r/1 -> Demux1/1
  q/1 -> Demux/1

== system Model_aircraft_simple/Trim/Gravity/Inertial_2_body1/Product of quaternions1/q3 ==
  q : Inport
  r : Inport  Port=2
  Demux : Demux
  Demux1 : Demux
  Product{,1..3} (4 alike) : Product  RndMeth=Zero
  Sum : Sum  Inputs=++-+
  q3 : Outport
  wires:
  Demux1/4 -> Product/2
  Demux1/3 -> Product1/2
  Demux1/1 -> Product3/2
  Demux1/2 -> Product2/2
  q/1 -> Demux/1
  r/1 -> Demux1/1
  Demux/1 -> Product/1
  Demux/2 -> Product1/1
  Demux/3 -> Product2/1
  Demux/4 -> Product3/1
  Product/1 -> Sum/1
  Product1/1 -> Sum/2
  Product3/1 -> Sum/4
  Sum/1 -> q3/1
  Product2/1 -> Sum/3

== system Model_aircraft_simple/Trim/Gravity/Inertial_2_body1/Product of quaternions2/q0 ==
  q : Inport
  r : Inport  Port=2
  Demux : Demux
  Demux1 : Demux
  Product{,1..3} (4 alike) : Product  RndMeth=Zero
  Sum : Sum  Inputs=+---
  q0 : Outport
  wires:
  q/1 -> Demux/1
  r/1 -> Demux1/1
  Demux/1 -> Product/1
  Demux1/1 -> Product/2
  Demux/2 -> Product1/1
  Demux1/2 -> Product1/2
  Demux/3 -> Product2/1
  Demux1/3 -> Product2/2
  Demux1/4 -> Product3/2
  Demux/4 -> Product3/1
  Product/1 -> Sum/1
  Product1/1 -> Sum/2
  Product3/1 -> Sum/4
  Sum/1 -> q0/1
  Product2/1 -> Sum/3

== system Model_aircraft_simple/Trim/Gravity/Inertial_2_body1/Product of quaternions2/q1 ==
  q : Inport
  r : Inport  Port=2
  Demux : Demux
  Demux1 : Demux
  Product{,1..3} (4 alike) : Product  RndMeth=Zero
  Sum : Sum  Inputs=+++-
  q1 : Outport
  wires:
  Product2/1 -> Sum/3
  Sum/1 -> q1/1
  Product3/1 -> Sum/4
  Product1/1 -> Sum/2
  Product/1 -> Sum/1
  Demux/4 -> Product3/1
  Demux/3 -> Product2/1
  Demux/2 -> Product1/1
  Demux/1 -> Product/1
  r/1 -> Demux1/1
  q/1 -> Demux/1
  Demux1/2 -> Product/2
  Demux1/1 -> Product1/2
  Demux1/4 -> Product2/2
  Demux1/3 -> Product3/2

== system Model_aircraft_simple/Trim/Gravity/Inertial_2_body1/Product of quaternions2/q2 ==
  q : Inport
  r : Inport  Port=2
  Demux : Demux
  Demux1 : Demux
  Product{,1..3} (4 alike) : Product  RndMeth=Zero
  Sum : Sum  Inputs=+-++
  q2 : Outport
  wires:
  q/1 -> Demux/1
  r/1 -> Demux1/1
  Demux/1 -> Product/1
  Demux/2 -> Product1/1
  Demux/3 -> Product2/1
  Demux/4 -> Product3/1
  Product/1 -> Sum/1
  Product1/1 -> Sum/2
  Product3/1 -> Sum/4
  Sum/1 -> q2/1
  Product2/1 -> Sum/3
  Demux1/3 -> Product/2
  Demux1/4 -> Product1/2
  Demux1/1 -> Product2/2
  Demux1/2 -> Product3/2

== system Model_aircraft_simple/Trim/Gravity/Inertial_2_body1/Product of quaternions2/q3 ==
  q : Inport
  r : Inport  Port=2
  Demux : Demux
  Demux1 : Demux
  Product{,1..3} (4 alike) : Product  RndMeth=Zero
  Sum : Sum  Inputs=++-+
  q3 : Outport
  wires:
  Product2/1 -> Sum/3
  Sum/1 -> q3/1
  Product3/1 -> Sum/4
  Product1/1 -> Sum/2
  Product/1 -> Sum/1
  Demux/4 -> Product3/1
  Demux/3 -> Product2/1
  Demux/2 -> Product1/1
  Demux/1 -> Product/1
  r/1 -> Demux1/1
  q/1 -> Demux/1
  Demux1/2 -> Product2/2
  Demux1/1 -> Product3/2
  Demux1/3 -> Product1/2
  Demux1/4 -> Product/2
